simulink model "AutoRS_Blatt_Simulink"  (R2022b)
settings: Solver=FixedStepAuto  StartTime=0.0  StopTime=100  FixedStep=1e-4  RelTol=1e-3
settings Model: Creator=Sebastian  LastModifiedBy=Sebastian

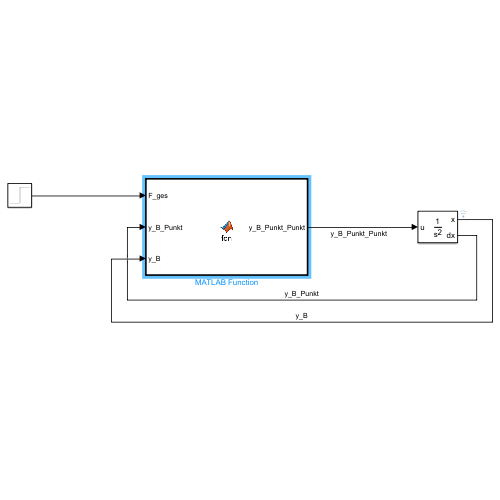
[thumbnail: Simulink's stored preview of the top-level diagram]
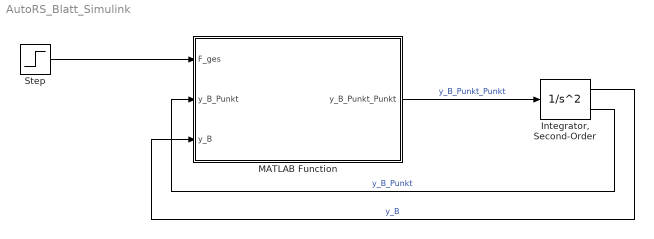
== system AutoRS_Blatt_Simulink ==
  "Integrator, Second-Order" : SecondOrderIntegrator  ICX=0
  MATLAB Function : MATLAB Function  TreatAsAtomicUnit=on
  Step : Step  Time=0  After=1e7  SampleTime=0
  wires:
  MATLAB Function/1(y_B_Punkt_Punkt) -> "Integrator, Second-Order"/1  "y_B_Punkt_Punkt"
  "Integrator, Second-Order"/2 -> MATLAB Function/2(y_B_Punkt)  "y_B_Punkt"
  "Integrator, Second-Order"/1 -> MATLAB Function/3(y_B)  "y_B"
  Step/1 -> MATLAB Function/1(F_ges)

== matlab function AutoRS_Blatt_Simulink/MATLAB Function ==
  data: F_ges input; y_B_Punkt input; y_B_Punkt_Punkt output; y_B input
function y_B_Punkt_Punkt = fcn(F_ges, y_B_Punkt, y_B)

    % KONSTANTEN
    c = Konstanten();
    
    % BERECHNUNG
    y_B_Punkt_Punkt = (F_ges-3*(c.d_B*y_B_Punkt)-3*(c.k_B*y_B))/(3*c.m_Bla);

end
